simulink model "test"  (R2018a)
settings: Solver=VariableStepAuto  StartTime=0.0  StopTime=10.0  RelTol=1e-3
settings Model: Creator=Abhishek Srivastava  LastModifiedBy=Abhishek Srivastava

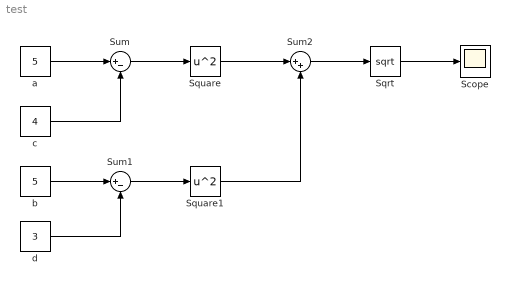
== system test ==
  Scope : Scope
  Sqrt : Sqrt  SaturateOnIntegerOverflow=on
  Square : Math  Operator=square  SaturateOnIntegerOverflow=on
  Square1 : Math  Operator=square  SaturateOnIntegerOverflow=on
  Sum : Sum  Inputs=|+-
  Sum1 : Sum  Inputs=|+-
  Sum2 : Sum  Inputs=|++
  a : Constant  Value=5
  b : Constant  Value=5
  c : Constant  Value=4
  d : Constant  Value=3
  wires:
  a/1 -> Sum/1
  c/1 -> Sum/2
  d/1 -> Sum1/2
  b/1 -> Sum1/1
  Sum1/1 -> Square1/1
  Sum/1 -> Square/1
  Square/1 -> Sum2/1
  Square1/1 -> Sum2/2
  Sum2/1 -> Sqrt/1
  Sqrt/1 -> Scope/1
